simulink model "VPNTZNN"  (R2024a)
settings: Solver=ode4  StartTime=0.0  StopTime=10.0  FixedStep=0.01  RelTol=1e-3
values from neighbouring files (symbols this model uses):
  alpha = 0.1    [setup.m]
  tau = 0.01    [setup.m]
  X0 = eye(2)    [setup.m]
undefined symbols (not defined in the file or in its folder): DiscIntNeverNeededParam, gaussian
libraries: simulink x1
settings Model: Creator=uli_2  LastModifiedBy=uli_2

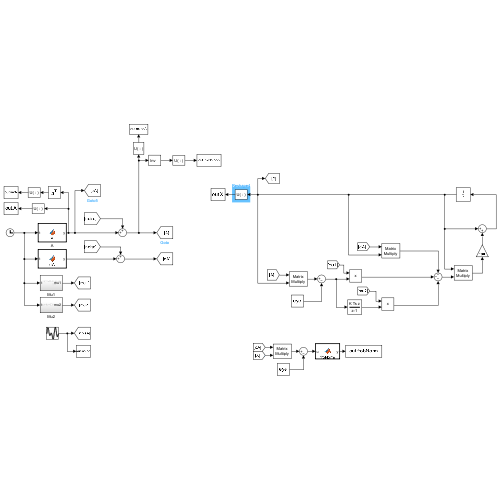
[thumbnail: Simulink's stored preview of the top-level diagram]
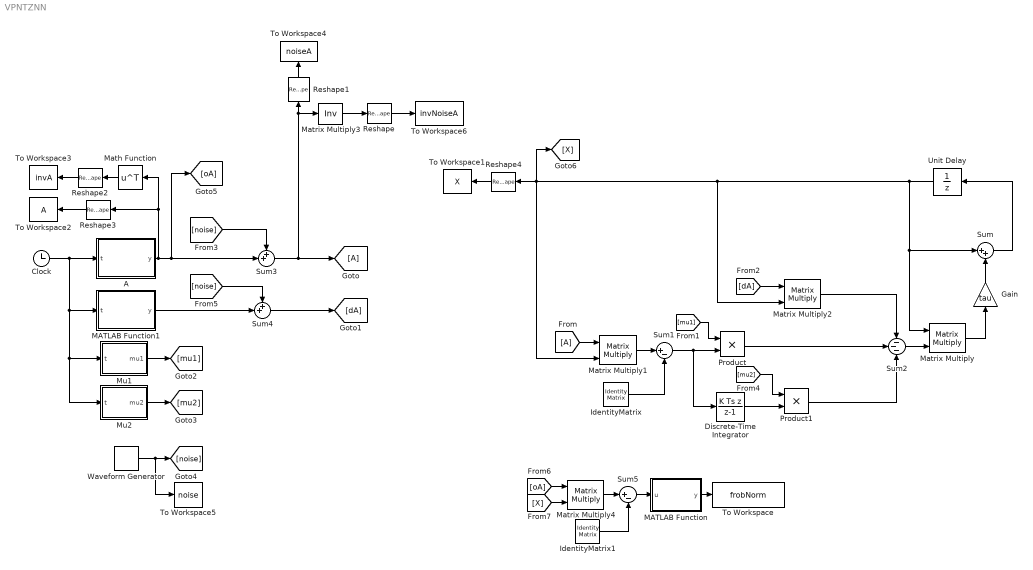
== system VPNTZNN ==
  A : MATLAB Function  TreatAsAtomicUnit=on
  Clock : Clock
  Discrete-Time Integrator : DiscreteIntegrator  IntegratorMethod=Integration: Backward Euler  InitialCondition=zeros(2)  SampleTime=-1  ICPrevOutput=DiscIntNeverNeededParam  ICPrevScaledInput=DiscIntNeverNeededParam
  From : From
  Gain : Gain  Gain=tau
  Goto : Goto
  IdentityMatrix : IdentityMatrix  OutputDimensions=2
  IdentityMatrix1 : IdentityMatrix  OutputDimensions=2
  MATLAB Function : MATLAB Function  TreatAsAtomicUnit=on
  MATLAB Function1 : MATLAB Function  TreatAsAtomicUnit=on
  Math Function : Math  Operator=transpose
  Matrix Multiply{,1..2,4} (4 alike) : Product  Multiplication=Matrix(*)
  Matrix Multiply3 : Product  Inputs=/  Multiplication=Matrix(*)
  Mu1 : Subsystem
  Mu2 : Subsystem
  Product : Product
  Product1 : Product
  Reshape{,1..4} (5 alike) : Reshape
  Sum : Sum  Inputs=|++
  Sum1 : Sum  Inputs=|+-
  Sum2 : Sum  Inputs=---
  Sum3 : Sum  Inputs=++|
  Sum4 : Sum  Inputs=++|
  Sum5 : Sum  Inputs=|+-
  To Workspace : ToWorkspace  VariableName=frobNorm  SaveFormat=Timeseries  SampleTime=-1
  To Workspace1 : ToWorkspace  VariableName=X  SaveFormat=Timeseries  SampleTime=-1
  To Workspace2 : ToWorkspace  VariableName=A  SaveFormat=Timeseries  SampleTime=-1
  To Workspace3 : ToWorkspace  VariableName=invA  SaveFormat=Timeseries  SampleTime=-1
  To Workspace4 : ToWorkspace  VariableName=noiseA  SaveFormat=Timeseries  SampleTime=-1
  To Workspace5 : ToWorkspace  VariableName=noise  SaveFormat=Timeseries  SampleTime=-1
  To Workspace6 : ToWorkspace  VariableName=invNoiseA  SaveFormat=Timeseries  SampleTime=-1
  Unit Delay : UnitDelay  InitialCondition=X0  SampleTime=-1  HasFrameUpgradeWarning=on
  Waveform Generator : simulink/Sources/Waveform Generator  OutMin=[]  OutMax=[]  OutDataTypeStr=double  SelectedSignal=1  Signals=0.1*gaussian(0,1,451)  BlockNames=MultiportSwitch_8127f67cd20a460  SampleTime=0.01
  wires:
  Unit Delay/1 -> Matrix Multiply2/2, Reshape4/1, [X], Matrix Multiply1/2, Matrix Multiply/1, Sum/1
  Gain/1 -> Sum/2
  Matrix Multiply/1 -> Gain/1
  Clock/1 -> Mu2/1(t), Mu1/1(t), MATLAB Function1/1(t), A/1(t)
  A/1(y) -> [oA], Sum3/2, Math Function/1, Reshape3/1
  Mu1/1(mu1) -> [mu1]
  Mu2/1(mu2) -> [mu2]
  From/1 -> Matrix Multiply1/1
  Matrix Multiply1/1 -> Sum1/1
  IdentityMatrix/1 -> Sum1/2
  Sum1/1 -> Discrete-Time Integrator/1, Product/2
  [mu1] -> Product/1
  Sum2/1 -> Matrix Multiply/2
  Sum/1 -> Unit Delay/1
  [dA] -> Matrix Multiply2/1
  Product/1 -> Sum2/2
  Matrix Multiply2/1 -> Sum2/1
  [mu2] -> Product1/1
  Product1/1 -> Sum2/3
  MATLAB Function/1(y) -> To Workspace/1
  Math Function/1 -> Reshape2/1
  Discrete-Time Integrator/1 -> Product1/2
  [noise] -> Sum3/1
  Waveform Generator/1 -> [noise], To Workspace5/1
  Sum3/1 -> Matrix Multiply3/1, Reshape1/1, Goto/1
  Matrix Multiply3/1 -> Reshape/1
  Sum4/1 -> [dA]
  MATLAB Function1/1(y) -> Sum4/2
  [noise] -> Sum4/1
  Matrix Multiply4/1 -> Sum5/1
  IdentityMatrix1/1 -> Sum5/2
  Sum5/1 -> MATLAB Function/1(u)
  [oA] -> Matrix Multiply4/1
  [X] -> Matrix Multiply4/2
  Reshape/1 -> To Workspace6/1
  Reshape1/1 -> To Workspace4/1
  Reshape2/1 -> To Workspace3/1
  Reshape3/1 -> To Workspace2/1
  Reshape4/1 -> To Workspace1/1

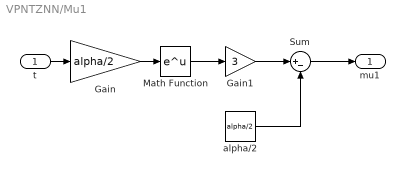
== system VPNTZNN/Mu1 ==
  t : Inport
  Gain : Gain  Gain=alpha/2
  Gain1 : Gain  Gain=3
  Math Function : Math
  Sum : Sum  Inputs=|+-
  alpha/2 : Constant  Value=alpha/2
  mu1 : Outport
  wires:
  Math Function/1 -> Gain1/1
  Gain/1 -> Math Function/1
  t/1 -> Gain/1
  Gain1/1 -> Sum/1
  Sum/1 -> mu1/1
  alpha/2/1 -> Sum/2

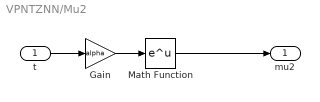
== system VPNTZNN/Mu2 ==
  t : Inport
  Gain : Gain  Gain=alpha
  Math Function : Math
  mu2 : Outport
  wires:
  t/1 -> Gain/1
  Gain/1 -> Math Function/1
  Math Function/1 -> mu2/1

== matlab function VPNTZNN/A ==
  data: t input; y output
function y = A(t)

y = [sin(t), cos(t); -cos(t), sin(t)];

== matlab function VPNTZNN/MATLAB Function ==
  data: u input; y output
function y = froNorm(u)
    y = norm(u, 'fro');

== matlab function VPNTZNN/MATLAB Function1 ==
  data: t input; y output
function y = dA(t)

y = [cos(t), -sin(t); sin(t), cos(t)];
